simulink model "QD2_DroneStack_PID_AM32ESC_R2022b"  (R2022b)
settings: Solver=ode1  StartTime=0.0  StopTime=inf  FixedStep=1/1000  RelTol=1e-3  EnableMultiTasking=on
InitFcn:
  | Motor_Mapping_7_Inch
model workspace (MAT data in the model file):
  target_system = 1
undefined symbols (not defined in the file): _Commander, _QDrone2, _Stabilizer, datetime, HIL, KT, lf, log_, log_QD2_, m, Motor_Matrix, n, qc_get_step_size, s, saved_data
libraries: quarc_library x170, simulink x35, simulink_extras x11
(part 4 of 7)

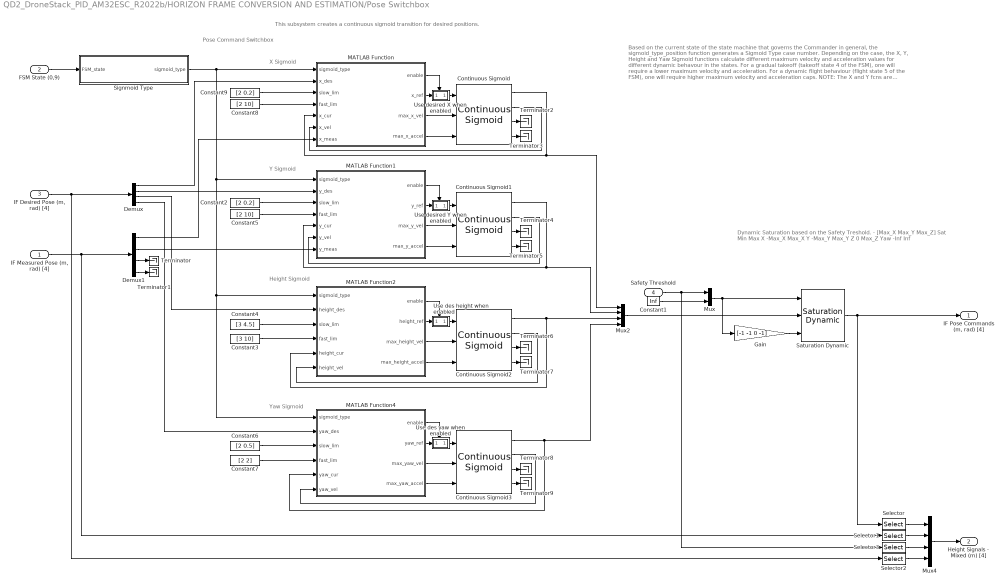
== system QD2_DroneStack_PID_AM32ESC_R2022b/HORIZON FRAME CONVERSION AND ESTIMATION/Pose Switchbox ==
  note: Dynamic Saturation based on the Safety Treshold. - [Max_X Max_Y Max_Z]
      |
      | Sat Min Max
      | X -Max_X Max_X
      | Y -Max_Y Max_Y
      | Z 0 Max_Z
      | Yaw -Inf Inf
  note: Based on the current state of the state machine that governs the Commander in general,
      | the sigmoid_type_position function generates a Sigmoid Type case number. Depending on
      | the case, the X, Y, Height and Yaw Sigmoid functions calculate different maximum velocity
      | and acceleration values for different dynamic behavour in the states.
      |
      | For a gradual takeoff (takeoff state 4 of the FSM), one will require a lower maximum velocity
      | and acceleration. For a dynamic flight behaviour (flight state 5 of the FSM), one will require
      | higher maximum velocity and acceleration caps.
      |
      | NOTE: The X and Y fcns are logically identical due to the generally symmetric X and Y behaviour.
      | The Z and Yaw fcns are different.
  note: This subsystem creates a continuous sigmoid transition for desired positions.
  note: Height Sigmoid
  note: Pose Command Switchbox
  note: X Sigmoid
  note: Yaw Sigmoid
  note: Y Sigmoid
  "IF Measured Pose (m, rad) [4]" : Inport
  FSM State (0,9) : Inport  Port=2
  "IF Desired Pose (m, rad) [4]" : Inport  Port=3
  Safety Threshold : Inport  Port=4
  Constant1 : Constant  Value=Inf
  Constant2 : Constant  Value=[2 0.2]
  Constant3 : Constant  Value=[3 10]
  Constant4 : Constant  Value=[3 4.5]
  Constant5 : Constant  Value=[2 10]
  Constant6 : Constant  Value=[2 0.5]
  Constant7 : Constant  Value=[2 2]
  Constant8 : Constant  Value=[2 10]
  Constant9 : Constant  Value=[2 0.2]
  Continuous Sigmoid{,1..3} (4 alike) : quarc_library/Sources/Sigmoids/Continuous Sigmoid  params_source=External (input ports)  max_velocity=2  max_acceleration=10  initial_position=0  initial_velocity=0  hold_off=0.5  input_sample_time=-1  output_sample_time=qc_get_step_size
      settings: SourceProductName=QUARC Targets
  Demux : Demux
  Demux1 : Demux
  Gain : Gain  Gain=[-1 -1 0 -1]
  MATLAB Function : MATLAB Function  TreatAsAtomicUnit=on
  MATLAB Function1 : MATLAB Function  TreatAsAtomicUnit=on
  MATLAB Function2 : MATLAB Function  TreatAsAtomicUnit=on
  MATLAB Function4 : MATLAB Function  TreatAsAtomicUnit=on
  Mux : Mux  Inputs=2
  Mux2 : Mux
  Mux4 : Mux
  Saturation Dynamic : simulink/Discontinuities/Saturation Dynamic  OutMin=[]  OutMax=[]  OutDataTypeStr=Inherit: Same as second input  OutDataType=fixdt(1, 16)  OutScaling=2^-10  DoSatur=off
  Selector : Selector  InputPortWidth=4  IndexOptions=Index vector (dialog)  Indices=[3]  OutputSizes=1
  Selector1 : Selector  InputPortWidth=4  IndexOptions=Index vector (dialog)  Indices=[3]  OutputSizes=1
  Selector2 : Selector  InputPortWidth=4  IndexOptions=Index vector (dialog)  Indices=[3]  OutputSizes=1
  Selector3 : Selector  InputPortWidth=3  IndexOptions=Index vector (dialog)  Indices=[3]  OutputSizes=1
  Signmoid Type : MATLAB Function  TreatAsAtomicUnit=on
  Terminator{,1..9} (10 alike) : Terminator
  Use des height when enabled : Subsystem  TreatAsAtomicUnit=on
  Use des yaw when enabled : Subsystem  TreatAsAtomicUnit=on
  Use desired X when enabled : Subsystem  TreatAsAtomicUnit=on
  Use desired Y when enabled : Subsystem  TreatAsAtomicUnit=on
  "IF Pose Commands (m, rad) [4]" : Outport  VectorParamsAs1DForOutWhenUnconnected=off
  Height Signals - Mixed (m) [4] : Outport  Port=2  VectorParamsAs1DForOutWhenUnconnected=off
  wires:
  Constant4/1 -> MATLAB Function2/3(slow_lim)
  Constant3/1 -> MATLAB Function2/4(fast_lim)
  Selector/1 -> Mux4/1
  Selector1/1 -> Mux4/2
  Selector2/1 -> Mux4/4
  Selector3/1 -> Mux4/3
  Safety Threshold/1 -> Mux/1, Selector3/1
  Mux/1 -> Saturation Dynamic/1, Gain/1
  Constant1/1 -> Mux/2
  Saturation Dynamic/1 -> "IF Pose Commands (m, rad) [4]"/1, Selector/1
  Mux2/1 -> Saturation Dynamic/2
  Mux4/1 -> Height Signals - Mixed (m) [4]/1
  Gain/1 -> Saturation Dynamic/3
  Demux/2 -> MATLAB Function1/2(y_des)
  Use desired Y when enabled/1(Out1) -> Continuous Sigmoid1/1
  Use desired X when enabled/1(Out1) -> Continuous Sigmoid/1
  MATLAB Function2/3(max_height_vel) -> Continuous Sigmoid2/2
  Continuous Sigmoid3/3 -> Terminator8/1
  Demux1/4 -> Terminator1/1
  MATLAB Function4/1(enable) -> Use des yaw when enabled/Enable
  Use des yaw when enabled/1(Out1) -> Continuous Sigmoid3/1
  Continuous Sigmoid1/2 -> MATLAB Function1/6(y_vel)
  Constant2/1 -> MATLAB Function1/3(slow_lim)
  Constant6/1 -> MATLAB Function4/3(slow_lim)
  Demux1/1 -> MATLAB Function/7(x_meas)
  MATLAB Function1/2(y_ref) -> Use desired Y when enabled/1(h_d (m) [1])
  Demux/3 -> MATLAB Function2/2(height_des)
  Constant7/1 -> MATLAB Function4/4(fast_lim)
  Continuous Sigmoid1/4 -> Terminator5/1
  MATLAB Function1/1(enable) -> Use desired Y when enabled/Enable
  Continuous Sigmoid2/4 -> Terminator7/1
  Demux1/3 -> Terminator/1
  Signmoid Type/1(sigmoid_type) -> MATLAB Function/1(sigmoid_type), MATLAB Function1/1(sigmoid_type), MATLAB Function2/1(sigmoid_type), MATLAB Function4/1(sigmoid_type)
  MATLAB Function/3(max_x_vel) -> Continuous Sigmoid/2
  MATLAB Function2/1(enable) -> Use des height when enabled/Enable
  Constant9/1 -> MATLAB Function/3(slow_lim)
  Continuous Sigmoid2/2 -> MATLAB Function2/6(height_vel)
  Continuous Sigmoid1/1 -> MATLAB Function1/5(y_cur), Mux2/2
  MATLAB Function4/4(max_yaw_accel) -> Continuous Sigmoid3/3
  Demux/1 -> MATLAB Function/2(x_des)
  MATLAB Function1/3(max_y_vel) -> Continuous Sigmoid1/2
  Continuous Sigmoid3/2 -> MATLAB Function4/6(yaw_vel)
  MATLAB Function2/2(height_ref) -> Use des height when enabled/1(h_d (m) [1])
  MATLAB Function/4(max_x_accel) -> Continuous Sigmoid/3
  Use des height when enabled/1(Out1) -> Continuous Sigmoid2/1
  Continuous Sigmoid2/3 -> Terminator6/1
  Demux/4 -> MATLAB Function4/2(yaw_des)
  MATLAB Function1/4(max_y_accel) -> Continuous Sigmoid1/3
  MATLAB Function/1(enable) -> Use desired X when enabled/Enable
  Continuous Sigmoid3/4 -> Terminator9/1
  MATLAB Function4/2(yaw_ref) -> Use des yaw when enabled/1(h_d (m) [1])
  FSM State (0,9)/1 -> Signmoid Type/1(FSM_state)
  MATLAB Function2/4(max_height_accel) -> Continuous Sigmoid2/3
  Continuous Sigmoid/4 -> Terminator3/1
  Continuous Sigmoid/3 -> Terminator2/1
  Continuous Sigmoid/1 -> MATLAB Function/5(x_cur), Mux2/1
  Continuous Sigmoid/2 -> MATLAB Function/6(x_vel)
  MATLAB Function/2(x_ref) -> Use desired X when enabled/1(h_d (m) [1])
  Continuous Sigmoid3/1 -> MATLAB Function4/5(yaw_cur), Mux2/4
  MATLAB Function4/3(max_yaw_vel) -> Continuous Sigmoid3/2
  Continuous Sigmoid2/1 -> MATLAB Function2/5(height_cur), Mux2/3
  Demux1/2 -> MATLAB Function1/7(y_meas)
  Continuous Sigmoid1/3 -> Terminator4/1
  "IF Measured Pose (m, rad) [4]"/1 -> Demux1/1, Selector1/1
  "IF Desired Pose (m, rad) [4]"/1 -> Demux/1, Selector2/1
  Constant5/1 -> MATLAB Function1/4(fast_lim)
  Constant8/1 -> MATLAB Function/4(fast_lim)

== system QD2_DroneStack_PID_AM32ESC_R2022b/QDrone 2 DAQ/Attitude Estimate from IMU Data ==
  IMU Data [12] : Inport
  For Each Subsystem - Iterate over IMU0 and IMU1 : Subsystem  TreatAsAtomicUnit=on
  Reshape into 2 columns for IMU0 and IMU1 : Reshape  OutputDimensionality=Customize  OutputDimensions=[6,2]
  Select Data for IMU0 : Selector  NumberOfDimensions=2  InputPortWidth=3  IndexOptions=Index vector (dialog),Index vector (dialog)  Indices=[1:9],[1]  OutputSizes=1,1
  Select Data for IMU1 : Selector  NumberOfDimensions=2  InputPortWidth=3  IndexOptions=Index vector (dialog),Index vector (dialog)  Indices=[1:9],[2]  OutputSizes=1,1
  "BF Estimated Attitude for IMU0 (rad, rad/s, rad/2^2) [9]" : Outport
  "BF Estimated Attitude for IMU1 (rad, rad/s, rad/2^2) [9]" : Outport  Port=2
  wires:
  IMU Data [12]/1 -> Reshape into 2 columns for IMU0 and IMU1/1
  Reshape into 2 columns for IMU0 and IMU1/1 -> For Each Subsystem - Iterate over IMU0 and IMU1/1(IMU Data [6xn])
  For Each Subsystem - Iterate over IMU0 and IMU1/1("BF Estimated Attitude (rad, rad/s, rad/2^2) [9xn]") -> Select Data for IMU1/1, Select Data for IMU0/1
  Select Data for IMU0/1 -> "BF Estimated Attitude for IMU0 (rad, rad/s, rad/2^2) [9]"/1
  Select Data for IMU1/1 -> "BF Estimated Attitude for IMU1 (rad, rad/s, rad/2^2) [9]"/1

== system QD2_DroneStack_PID_AM32ESC_R2022b/QDrone 2 DAQ/Choose Motor Telemetry ==
  enable telemetry : Inport
  Bias1 : Bias  Bias=0:3  SaturateOnIntegerOverflow=off
  Constant1 : Constant  Value="[0 0 0 0; 1 0 0 0; 0 0 0 0; 0 1 0 0; 0 0 0 0; 0 0 1 0; 0 0 0 0;  0 0 0 1]"
  Constant2 : Constant  Value=8
  Gain : Gain  Gain=.7
  MATLAB Function : MATLAB Function  TreatAsAtomicUnit=on
  Selector : Selector  NumberOfDimensions=2  IndexMode=Zero-based  InputPortWidth=3  IndexOptions=Index vector (port),Select all  Indices=[1 3],1  OutputSizes=1,1
  Telemetry : Scope
  Zero-Order Hold1 : ZeroOrderHold  SampleTime=-1
  Motor telemetry select : Outport
  Motor telemetry index : Outport  Port=2
  wires:
  Gain/1 -> Bias1/1
  Bias1/1 -> Telemetry/1
  MATLAB Function/1(idx) -> Zero-Order Hold1/1
  Zero-Order Hold1/1 -> Selector/2, Motor telemetry index/1
  enable telemetry/1 -> MATLAB Function/1(enable)
  Selector/1 -> Motor telemetry select/1, Gain/1
  Constant1/1 -> Selector/1
  Constant2/1 -> MATLAB Function/2(n)

== system QD2_DroneStack_PID_AM32ESC_R2022b/QDrone 2 DAQ/Construct ESC Speed ==
  ESC Data In [4] : Inport
  ESC Channel Select : Inport  Port=2
  For Each Subsystem - Construct ESC Signal : Subsystem  TreatAsAtomicUnit=on
  Memory : Memory  InitialCondition=zeros(1,4)
  ESC Data Out [4] : Outport
  wires:
  For Each Subsystem - Construct ESC Signal/1(ESC Data Out [4]) -> ESC Data Out [4]/1, Memory/1
  Memory/1 -> For Each Subsystem - Construct ESC Signal/3(ESC Previous Data [4])
  ESC Data In [4]/1 -> For Each Subsystem - Construct ESC Signal/1(ESC Data In [4])
  ESC Channel Select/1 -> For Each Subsystem - Construct ESC Signal/2(ESC Channel)

== system QD2_DroneStack_PID_AM32ESC_R2022b/QDrone 2 DAQ/Construct ESC Temperature ==
  ESC Data In [4] : Inport
  ESC Channel Select : Inport  Port=2
  For Each Subsystem - Construct ESC Signal : Subsystem  TreatAsAtomicUnit=on
  Memory : Memory  InitialCondition=zeros(1,4)
  ESC Data Out [4] : Outport
  wires:
  For Each Subsystem - Construct ESC Signal/1(ESC Data Out [4]) -> ESC Data Out [4]/1, Memory/1
  Memory/1 -> For Each Subsystem - Construct ESC Signal/3(ESC Previous Data [4])
  ESC Data In [4]/1 -> For Each Subsystem - Construct ESC Signal/1(ESC Data In [4])
  ESC Channel Select/1 -> For Each Subsystem - Construct ESC Signal/2(ESC Channel)

== system QD2_DroneStack_PID_AM32ESC_R2022b/QDrone 2 DAQ/Construct ESC Voltage ==
  ESC Data In [4] : Inport
  ESC Channel Select : Inport  Port=2
  For Each Subsystem - Construct ESC Signal : Subsystem  TreatAsAtomicUnit=on
  Memory : Memory  InitialCondition=zeros(1,4)
  ESC Data Out [4] : Outport
  wires:
  ESC Channel Select/1 -> For Each Subsystem - Construct ESC Signal/2(ESC Channel)
  ESC Data In [4]/1 -> For Each Subsystem - Construct ESC Signal/1(ESC Data In [4])
  Memory/1 -> For Each Subsystem - Construct ESC Signal/3(ESC Previous Data [4])
  For Each Subsystem - Construct ESC Signal/1(ESC Data Out [4]) -> Memory/1, ESC Data Out [4]/1

== system QD2_DroneStack_PID_AM32ESC_R2022b/QDrone 2 DAQ/Detect ESC Problems ==
  ESC Telemetry Enabled : Inport
  ESC Channel Request [4] : Inport  Port=2
  ESC Channel Reported [4] : Inport  Port=3
  AND : Logic  IconShape=distinctive  AllPortsSameDT=off  OutDataTypeStr=boolean
  Compare To Constant : simulink/Logic and Bit Operations/Compare To Constant  relop=>=  const=20  OutDataTypeStr=boolean
  Constant : Constant  Value=200
  Delay{,1..3} (4 alike) : Delay
  Demux{,1..2,8} (4 alike) : Demux
  ESC Channel Mismatrch : Scope  NumInputPorts=4
  ESC Channel Mismatrch Count : Scope  NumInputPorts=4
  ESC Channel Selection Index : Scope  NumInputPorts=4
  For Each Subsystem : Subsystem  TreatAsAtomicUnit=on
  MATLAB Function : MATLAB Function  TreatAsAtomicUnit=on
  Mux : Mux
  Mux{1..4} (4 alike) : Mux  Inputs=2
  ESC Comm Problem [4] : Outport
  wires:
  ESC Channel Reported [4]/1 -> Demux2/1, For Each Subsystem/2(Channel Reported [4])
  Demux/1 -> Delay3/1
  Demux/2 -> Delay2/1
  Demux/3 -> Delay1/1
  Demux/4 -> Delay/1
  ESC Channel Request [4]/1 -> Demux/1
  Delay2/1 -> Mux2/1, Mux/2
  Delay3/1 -> Mux/1, Mux1/1
  Delay1/1 -> Mux3/1, Mux/3
  Delay/1 -> Mux4/1, Mux/4
  Mux/1 -> For Each Subsystem/1(Channel Requested [4])
  For Each Subsystem/1(mismatched [4]) -> AND/1
  AND/1 -> MATLAB Function/1(u), Demux8/1
  Demux8/2 -> ESC Channel Mismatrch/3
  Demux8/1 -> ESC Channel Mismatrch/4
  Demux8/3 -> ESC Channel Mismatrch/2
  Demux8/4 -> ESC Channel Mismatrch/1
  Constant/1 -> MATLAB Function/2(buffer_size)
  Demux1/4 -> ESC Channel Mismatrch Count/1
  Demux1/3 -> ESC Channel Mismatrch Count/2
  Demux1/1 -> ESC Channel Mismatrch Count/4
  Demux1/2 -> ESC Channel Mismatrch Count/3
  MATLAB Function/1(n) -> Compare To Constant/1, Demux1/1
  Compare To Constant/1 -> ESC Comm Problem [4]/1
  ESC Telemetry Enabled/1 -> AND/2
  Demux2/1 -> Mux1/2
  Demux2/2 -> Mux2/2
  Demux2/3 -> Mux3/2
  Demux2/4 -> Mux4/2
  Mux4/1 -> ESC Channel Selection Index/1
  Mux3/1 -> ESC Channel Selection Index/2
  Mux2/1 -> ESC Channel Selection Index/3
  Mux1/1 -> ESC Channel Selection Index/4

== system QD2_DroneStack_PID_AM32ESC_R2022b/QDrone 2 DAQ/Enabled Subsystem - Write ESC Commands ==
  DShot Raw [4] : Inport
  Enable : EnablePort
  HIL Write PWM : quarc_library/Data Acquisition/Generic/Immediate I//O/HIL Write PWM  object_name=HIL-1  channels=[0:3]  sample_time=-1  active=off  vector_input=on
      settings: AttributesFormatString=(%<object_name>)  SourceProductName=QUARC Targets
  wires:
  DShot Raw [4]/1 -> HIL Write PWM/1

== system QD2_DroneStack_PID_AM32ESC_R2022b/QDrone 2 DAQ/Generate LED Pattern ==
  ESC States : Inport
  Blue Blue : Constant  Value=[0 0 1 0 0 1]
  Green Green : Constant  Value=[0 1 0 0 1 0]
  LED OFF : Constant  Value=[ 0 0 0 0 0 0]
  Multiport Switch : MultiPortSwitch  DataPortOrder=Specify indices  DataPortIndices={0,1,2,3,4,5,77,88,99}  DataPortForDefault=Additional data port  DiagnosticForDefault=Warning  SaturateOnIntegerOverflow=off  InputSameDT=off
  Red Blue : Constant  Value="[ 1 0 0 0 0 1   ]"
  Red Red : Constant  Value=[ 1 0 0 1 0 0]
  Red Yellow : Constant  Value="[ 1 0 0 1 1 0  ]"
  Yellow Blue : Constant  Value="[ 1 1 0 0 0 1  ]"
  Yellow Green : Constant  Value="[ 1 1 0 0 1 0  ]"
  Yellow Red : Constant  Value="[ 1 1 0 1 0 0  ]"
  Yellow Yellow : Constant  Value="[ 1 1 0 1 1 0  ]"
  LED Command : Outport
  wires:
  Multiport Switch/1 -> LED Command/1
  ESC States/1 -> Multiport Switch/1
  Blue Blue/1 -> Multiport Switch/4
  Red Red/1 -> Multiport Switch/10
  Yellow Yellow/1 -> Multiport Switch/2
  Red Blue/1 -> Multiport Switch/9
  Yellow Blue/1 -> Multiport Switch/8
  LED OFF/1 -> Multiport Switch/11
  Green Green/1 -> Multiport Switch/7
  Yellow Green/1 -> Multiport Switch/3
  Yellow Red/1 -> Multiport Switch/5
  Red Yellow/1 -> Multiport Switch/6

== system QD2_DroneStack_PID_AM32ESC_R2022b/QDrone 2 DAQ/Monitor Battery Level ==
  note: Monitor Battery Level.
      | Flag Low Battery Error if
      | Battery level dips below
      | threshold for specified
      | threshold time period.
  Battery (V) : Inport
  AND : Logic  IconShape=distinctive  AllPortsSameDT=off  OutDataTypeStr=boolean
  Battery Low Time Threshold (s) : Constant  Value=0.3
  Constant : Constant  Value=0.5
  Data Type Conversion : DataTypeConversion  SaturateOnIntegerOverflow=off  RndMeth=Floor
  Data Type Conversion1 : DataTypeConversion  SaturateOnIntegerOverflow=off  RndMeth=Floor
  Greater than minimum expected voltage (Valid Battery Reading) : simulink/Logic and Bit Operations/Compare To Constant  relop=>  const=0.5  OutDataTypeStr=boolean
  Less than minimum threshold voltage (Battery level too low) : simulink/Logic and Bit Operations/Compare To Constant  relop=<=  const=14  OutDataTypeStr=boolean
  Terminator : Terminator
  Threshold : quarc_library/Discontinuities/Threshold  operator=>=  param_src=External input port  threshold=0  duration=0
      settings: SourceProductName=QUARC Targets
  Triggered Subsystem - Latching Flag : Subsystem  TreatAsAtomicUnit=on
  Low Battery : Outport
  wires:
  Battery (V)/1 -> Less than minimum threshold voltage (Battery level too low)/1, Greater than minimum expected voltage (Valid Battery Reading)/1
  Less than minimum threshold voltage (Battery level too low)/1 -> AND/2
  Greater than minimum expected voltage (Valid Battery Reading)/1 -> AND/1
  AND/1 -> Data Type Conversion/1
  Constant/1 -> Threshold/2
  Battery Low Time Threshold (s)/1 -> Threshold/3
  Data Type Conversion/1 -> Threshold/1
  Threshold/2 -> Terminator/1
  Threshold/1 -> Triggered Subsystem - Latching Flag/Trigger
  Triggered Subsystem - Latching Flag/1(Out1) -> Data Type Conversion1/1
  Data Type Conversion1/1 -> Low Battery/1

== system QD2_DroneStack_PID_AM32ESC_R2022b/QDrone 2 DAQ/Sensor Failure Monitoring ==
  note: Check if any of the IMU signal lines have "flatlined"
      | i.e., remain at exactly 0 value for 1 second or more
  IMU Data [12] : Inport
  Model Time : Inport  Port=2
  AND : Logic  IconShape=distinctive  AllPortsSameDT=off  OutDataTypeStr=boolean
  Compare : quarc_library/Logic Operations/Compare  operator=>=  output_data_type=boolean
      settings: SourceProductName=QUARC Targets
  Constant1 : Constant
  Constant2 : Constant  Value=0
  Demux : Demux  Outputs=12
  OR : Logic  Operator=OR  Inputs=12  AllPortsSameDT=off  OutDataTypeStr=boolean
  Terminator{,1..11} (12 alike) : Terminator
  Threshold{,1..11} (12 alike) : quarc_library/Discontinuities/Threshold  operator===  param_src=External input port  threshold=0  duration=1
      settings: SourceProductName=QUARC Targets
  Sensor Fault : Outport
  wires:
  Model Time/1 -> Compare/1
  Constant1/1 -> Threshold1/3, Threshold2/3, Threshold3/3, Threshold5/3, Threshold6/3, Threshold7/3, Threshold8/3, Threshold9/3, Threshold10/3, Threshold11/3, Threshold4/3, Threshold/3, Compare/2
  Demux/1 -> Threshold/1
  Demux/2 -> Threshold1/1
  Constant2/1 -> Threshold1/2, Threshold2/2, Threshold3/2, Threshold4/2, Threshold5/2, Threshold6/2, Threshold7/2, Threshold8/2, Threshold9/2, Threshold10/2, Threshold11/2, Threshold/2
  IMU Data [12]/1 -> Demux/1
  Demux/3 -> Threshold2/1
  Demux/4 -> Threshold3/1
  Demux/5 -> Threshold4/1
  Demux/6 -> Threshold5/1
  Demux/7 -> Threshold6/1
  Demux/8 -> Threshold7/1
  Demux/9 -> Threshold8/1
  Demux/10 -> Threshold9/1
  Demux/11 -> Threshold10/1
  Demux/12 -> Threshold11/1
  Threshold/1 -> OR/1
  Threshold1/1 -> OR/2
  Threshold2/1 -> OR/3
  Threshold3/1 -> OR/4
  Threshold4/1 -> OR/5
  Threshold5/1 -> OR/6
  Threshold6/1 -> OR/7
  Threshold7/1 -> OR/8
  Threshold8/1 -> OR/9
  Threshold9/1 -> OR/10
  Threshold10/1 -> OR/11
  Threshold11/1 -> OR/12
  Threshold/2 -> Terminator/1
  Threshold1/2 -> Terminator1/1
  Threshold2/2 -> Terminator2/1
  Threshold3/2 -> Terminator3/1
  Threshold4/2 -> Terminator4/1
  Threshold5/2 -> Terminator5/1
  Threshold6/2 -> Terminator6/1
  Threshold7/2 -> Terminator7/1
  Threshold8/2 -> Terminator8/1
  Threshold9/2 -> Terminator9/1
  Threshold10/2 -> Terminator10/1
  Threshold11/2 -> Terminator11/1
  Compare/1 -> AND/1
  OR/1 -> AND/2
  AND/1 -> Sensor Fault/1

== system QD2_DroneStack_PID_AM32ESC_R2022b/QDrone 2 DAQ/Timing Monitors ==
  note: Base Model Rate (1kHz)
  note: Optical Flow Rate (100 Hz)
  note: ToF Range Rate (25 Hz)
  Computation Time : quarc_library/Sources/Time/Computation Time  sample_time=qc_get_step_size  use_model=on  use_cpu_time=off
  Computation Time1 : quarc_library/Sources/Time/Computation Time  sample_time=0.01  use_model=on  use_cpu_time=off
  Computation Time2 : quarc_library/Sources/Time/Computation Time  sample_time=0.04  use_model=on  use_cpu_time=off
  Mux : Mux  Inputs=2
  Mux1 : Mux  Inputs=2
  Mux2 : Mux  Inputs=2
  Mux3 : Mux  Inputs=3
  Rate Transition{,1..3} (4 alike) : RateTransition
  Sample Time : quarc_library/Sources/Time/Sample Time  Priority=-99  sample_time=qc_get_step_size
  Sample Time1 : quarc_library/Sources/Time/Sample Time  Priority=-99  sample_time=0.01
  Sample Time2 : quarc_library/Sources/Time/Sample Time  Priority=-99  sample_time=0.04
  Timing Check : Scope  NumInputPorts=3
  Timings : Outport
  wires:
  Computation Time/1 -> Mux/1
  Sample Time/1 -> Mux/2
  Sample Time1/1 -> Rate Transition1/1
  Computation Time1/1 -> Rate Transition/1
  Computation Time2/1 -> Rate Transition2/1
  Sample Time2/1 -> Rate Transition3/1
  Mux1/1 -> Mux3/2, Timing Check/2
  Mux/1 -> Timing Check/1, Mux3/1
  Mux2/1 -> Timing Check/3, Mux3/3
  Mux3/1 -> Timings/1
  Rate Transition/1 -> Mux1/1
  Rate Transition1/1 -> Mux1/2
  Rate Transition2/1 -> Mux2/1
  Rate Transition3/1 -> Mux2/2

== system QD2_DroneStack_PID_AM32ESC_R2022b/QDrone 2 DAQ - OLD/Attitude Estimate from IMU Data ==
  IMU Data [12] : Inport
  For Each Subsystem - Iterate over IMU0 and IMU1 : Subsystem  TreatAsAtomicUnit=on
  Reshape into 2 columns for IMU0 and IMU1 : Reshape  OutputDimensionality=Customize  OutputDimensions=[6,2]
  Select Data for IMU0 : Selector  NumberOfDimensions=2  InputPortWidth=3  IndexOptions=Index vector (dialog),Index vector (dialog)  Indices=[1:9],[1]  OutputSizes=1,1
  Select Data for IMU1 : Selector  NumberOfDimensions=2  InputPortWidth=3  IndexOptions=Index vector (dialog),Index vector (dialog)  Indices=[1:9],[2]  OutputSizes=1,1
  "BF Estimated Attitude for IMU0 (rad, rad/s, rad/2^2) [9]" : Outport
  "BF Estimated Attitude for IMU1 (rad, rad/s, rad/2^2) [9]" : Outport  Port=2
  wires:
  IMU Data [12]/1 -> Reshape into 2 columns for IMU0 and IMU1/1
  Reshape into 2 columns for IMU0 and IMU1/1 -> For Each Subsystem - Iterate over IMU0 and IMU1/1(IMU Data [6xn])
  For Each Subsystem - Iterate over IMU0 and IMU1/1("BF Estimated Attitude (rad, rad/s, rad/2^2) [9xn]") -> Select Data for IMU1/1, Select Data for IMU0/1
  Select Data for IMU0/1 -> "BF Estimated Attitude for IMU0 (rad, rad/s, rad/2^2) [9]"/1
  Select Data for IMU1/1 -> "BF Estimated Attitude for IMU1 (rad, rad/s, rad/2^2) [9]"/1

== system QD2_DroneStack_PID_AM32ESC_R2022b/QDrone 2 DAQ - OLD/Choose Motor Telemetry ==
  enable telemetry : Inport
  Bias1 : Bias  Bias=0:3  SaturateOnIntegerOverflow=off
  Constant1 : Constant  Value=[0 0 0 0; 0 0 0 1; 0 0 0 0; 0 0 1 0; 0 0 0 0; 0 1 0 0; 0 0 0 0; 1 0 0 0]
  Constant2 : Constant  Value=8
  Gain : Gain  Gain=.7
  MATLAB Function : MATLAB Function  TreatAsAtomicUnit=on
  Selector : Selector  NumberOfDimensions=2  IndexMode=Zero-based  InputPortWidth=3  IndexOptions=Index vector (port),Select all  Indices=[1 3],1  OutputSizes=1,1
  Telemetry : Scope
  Zero-Order Hold1 : ZeroOrderHold  SampleTime=-1
  Motor telemetry select : Outport
  Motor telemetry index : Outport  Port=2
  wires:
  Gain/1 -> Bias1/1
  Bias1/1 -> Telemetry/1
  MATLAB Function/1(idx) -> Zero-Order Hold1/1
  Zero-Order Hold1/1 -> Selector/2, Motor telemetry index/1
  enable telemetry/1 -> MATLAB Function/1(enable)
  Selector/1 -> Motor telemetry select/1, Gain/1
  Constant1/1 -> Selector/1
  Constant2/1 -> MATLAB Function/2(n)

== system QD2_DroneStack_PID_AM32ESC_R2022b/QDrone 2 DAQ - OLD/Construct ESC Speed ==
  ESC Data In [4] : Inport
  ESC Channel Select : Inport  Port=2
  For Each Subsystem - Construct ESC Signal : Subsystem  TreatAsAtomicUnit=on
  Memory : Memory  InitialCondition=zeros(1,4)
  ESC Data Out [4] : Outport
  wires:
  For Each Subsystem - Construct ESC Signal/1(ESC Data Out [4]) -> ESC Data Out [4]/1, Memory/1
  Memory/1 -> For Each Subsystem - Construct ESC Signal/3(ESC Previous Data [4])
  ESC Data In [4]/1 -> For Each Subsystem - Construct ESC Signal/1(ESC Data In [4])
  ESC Channel Select/1 -> For Each Subsystem - Construct ESC Signal/2(ESC Channel)

== system QD2_DroneStack_PID_AM32ESC_R2022b/QDrone 2 DAQ - OLD/Construct ESC Temperature ==
  ESC Data In [4] : Inport
  ESC Channel Select : Inport  Port=2
  For Each Subsystem - Construct ESC Signal : Subsystem  TreatAsAtomicUnit=on
  Memory : Memory  InitialCondition=zeros(1,4)
  ESC Data Out [4] : Outport
  wires:
  For Each Subsystem - Construct ESC Signal/1(ESC Data Out [4]) -> ESC Data Out [4]/1, Memory/1
  Memory/1 -> For Each Subsystem - Construct ESC Signal/3(ESC Previous Data [4])
  ESC Data In [4]/1 -> For Each Subsystem - Construct ESC Signal/1(ESC Data In [4])
  ESC Channel Select/1 -> For Each Subsystem - Construct ESC Signal/2(ESC Channel)

== system QD2_DroneStack_PID_AM32ESC_R2022b/QDrone 2 DAQ - OLD/Construct ESC Voltage ==
  ESC Data In [4] : Inport
  ESC Channel Select : Inport  Port=2
  For Each Subsystem - Construct ESC Signal : Subsystem  TreatAsAtomicUnit=on
  Memory : Memory  InitialCondition=zeros(1,4)
  ESC Data Out [4] : Outport
  wires:
  ESC Channel Select/1 -> For Each Subsystem - Construct ESC Signal/2(ESC Channel)
  ESC Data In [4]/1 -> For Each Subsystem - Construct ESC Signal/1(ESC Data In [4])
  Memory/1 -> For Each Subsystem - Construct ESC Signal/3(ESC Previous Data [4])
  For Each Subsystem - Construct ESC Signal/1(ESC Data Out [4]) -> Memory/1, ESC Data Out [4]/1

== system QD2_DroneStack_PID_AM32ESC_R2022b/QDrone 2 DAQ - OLD/Detect ESC Problems ==
  ESC Telemetry Enabled : Inport
  ESC Channel Request [4] : Inport  Port=2
  ESC Channel Reported [4] : Inport  Port=3
  AND : Logic  IconShape=distinctive  AllPortsSameDT=off  OutDataTypeStr=boolean
  Compare To Constant : simulink/Logic and Bit Operations/Compare To Constant  relop=>=  const=10  OutDataTypeStr=boolean
  Constant : Constant  Value=100
  Delay{,1..3} (4 alike) : Delay
  Demux : Demux
  Demux1 : Demux
  Demux8 : Demux
  ESC Channel Mismatrch : Scope  NumInputPorts=4
  ESC Channel Mismatrch Count : Scope  NumInputPorts=4
  For Each Subsystem : Subsystem  TreatAsAtomicUnit=on
  MATLAB Function : MATLAB Function  TreatAsAtomicUnit=on
  Mux : Mux
  ESC Comm Problem [4] : Outport
  wires:
  ESC Channel Reported [4]/1 -> For Each Subsystem/2(Channel Reported [4])
  Demux/1 -> Delay3/1
  Demux/2 -> Delay2/1
  Demux/3 -> Delay1/1
  Demux/4 -> Delay/1
  ESC Channel Request [4]/1 -> Demux/1
  Delay2/1 -> Mux/2
  Delay3/1 -> Mux/1
  Delay1/1 -> Mux/3
  Delay/1 -> Mux/4
  Mux/1 -> For Each Subsystem/1(Channel Requested [4])
  For Each Subsystem/1(mismatched [4]) -> AND/1
  AND/1 -> MATLAB Function/1(u), Demux8/1
  Demux8/2 -> ESC Channel Mismatrch/3
  Demux8/1 -> ESC Channel Mismatrch/4
  Demux8/3 -> ESC Channel Mismatrch/2
  Demux8/4 -> ESC Channel Mismatrch/1
  Constant/1 -> MATLAB Function/2(buffer_size)
  Demux1/4 -> ESC Channel Mismatrch Count/1
  Demux1/3 -> ESC Channel Mismatrch Count/2
  Demux1/1 -> ESC Channel Mismatrch Count/4
  Demux1/2 -> ESC Channel Mismatrch Count/3
  MATLAB Function/1(n) -> Compare To Constant/1, Demux1/1
  Compare To Constant/1 -> ESC Comm Problem [4]/1
  ESC Telemetry Enabled/1 -> AND/2

== system QD2_DroneStack_PID_AM32ESC_R2022b/QDrone 2 DAQ - OLD/Enabled Subsystem - Write ESC Commands ==
  DShot Raw [4] : Inport
  Enable : EnablePort
  HIL Write PWM : quarc_library/Data Acquisition/Generic/Immediate I//O/HIL Write PWM  object_name=HIL-1  channels=[0:3]  sample_time=-1  active=off  vector_input=on
      settings: AttributesFormatString=(%<object_name>)  SourceProductName=QUARC Targets
  wires:
  DShot Raw [4]/1 -> HIL Write PWM/1

== system QD2_DroneStack_PID_AM32ESC_R2022b/QDrone 2 DAQ - OLD/Generate LED Pattern ==
  ESC States : Inport
  Blue Blue : Constant  Value=[0 0 1 0 0 1]
  Green Green : Constant  Value=[0 1 0 0 1 0]
  LED OFF : Constant  Value=[ 0 0 0 0 0 0]
  Multiport Switch : MultiPortSwitch  DataPortOrder=Specify indices  DataPortIndices={0,1,2,3,4,5,77,88,99}  DataPortForDefault=Additional data port  DiagnosticForDefault=Warning  SaturateOnIntegerOverflow=off  InputSameDT=off
  Red Blue : Constant  Value="[ 1 0 0 0 0 1   ]"
  Red Red : Constant  Value=[ 1 0 0 1 0 0]
  Red Yellow : Constant  Value="[ 1 0 0 1 1 0  ]"
  Yellow Blue : Constant  Value="[ 1 1 0 0 0 1  ]"
  Yellow Green : Constant  Value="[ 1 1 0 0 1 0  ]"
  Yellow Red : Constant  Value="[ 1 1 0 1 0 0  ]"
  Yellow Yellow : Constant  Value="[ 1 1 0 1 1 0  ]"
  LED Command : Outport
  wires:
  Multiport Switch/1 -> LED Command/1
  ESC States/1 -> Multiport Switch/1
  Blue Blue/1 -> Multiport Switch/4
  Red Red/1 -> Multiport Switch/10
  Yellow Yellow/1 -> Multiport Switch/2
  Red Blue/1 -> Multiport Switch/9
  Yellow Blue/1 -> Multiport Switch/8
  LED OFF/1 -> Multiport Switch/11
  Green Green/1 -> Multiport Switch/7
  Yellow Green/1 -> Multiport Switch/3
  Yellow Red/1 -> Multiport Switch/5
  Red Yellow/1 -> Multiport Switch/6

== system QD2_DroneStack_PID_AM32ESC_R2022b/QDrone 2 DAQ - OLD/Monitor Battery Level ==
  note: Monitor Battery Level.
      | Flag Low Battery Error if
      | Battery level dips below
      | threshold for specified
      | threshold time period.
  Battery (V) : Inport
  AND : Logic  IconShape=distinctive  AllPortsSameDT=off  OutDataTypeStr=boolean
  Battery Low Time Threshold (s) : Constant  Value=0.3
  Constant : Constant  Value=0.5
  Data Type Conversion : DataTypeConversion  SaturateOnIntegerOverflow=off  RndMeth=Floor
  Data Type Conversion1 : DataTypeConversion  SaturateOnIntegerOverflow=off  RndMeth=Floor
  Greater than minimum expected voltage (Valid Battery Reading) : simulink/Logic and Bit Operations/Compare To Constant  relop=>  const=0.5  OutDataTypeStr=boolean
  Less than minimum threshold voltage (Battery level too low) : simulink/Logic and Bit Operations/Compare To Constant  relop=<=  const=14  OutDataTypeStr=boolean
  Terminator : Terminator
  Threshold : quarc_library/Discontinuities/Threshold  operator=>=  param_src=External input port  threshold=0  duration=0
      settings: SourceProductName=QUARC Targets
  Triggered Subsystem - Latching Flag : Subsystem  TreatAsAtomicUnit=on
  Low Battery : Outport
  wires:
  Battery (V)/1 -> Less than minimum threshold voltage (Battery level too low)/1, Greater than minimum expected voltage (Valid Battery Reading)/1
  Less than minimum threshold voltage (Battery level too low)/1 -> AND/2
  Greater than minimum expected voltage (Valid Battery Reading)/1 -> AND/1
  AND/1 -> Data Type Conversion/1
  Constant/1 -> Threshold/2
  Battery Low Time Threshold (s)/1 -> Threshold/3
  Data Type Conversion/1 -> Threshold/1
  Threshold/2 -> Terminator/1
  Threshold/1 -> Triggered Subsystem - Latching Flag/Trigger
  Triggered Subsystem - Latching Flag/1(Out1) -> Data Type Conversion1/1
  Data Type Conversion1/1 -> Low Battery/1

== system QD2_DroneStack_PID_AM32ESC_R2022b/QDrone 2 DAQ - OLD/Sensor Failure Monitoring ==
  note: Check if any of the IMU signal lines have "flatlined"
      | i.e., remain at exactly 0 value for 1 second or more
  IMU Data [12] : Inport
  Model Time : Inport  Port=2
  AND : Logic  IconShape=distinctive  AllPortsSameDT=off  OutDataTypeStr=boolean
  Compare : quarc_library/Logic Operations/Compare  operator=>=  output_data_type=boolean
      settings: SourceProductName=QUARC Targets
  Constant1 : Constant
  Constant2 : Constant  Value=0
  Demux : Demux  Outputs=12
  OR : Logic  Operator=OR  Inputs=12  AllPortsSameDT=off  OutDataTypeStr=boolean
  Terminator{,1..11} (12 alike) : Terminator
  Threshold{,1..11} (12 alike) : quarc_library/Discontinuities/Threshold  operator===  param_src=External input port  threshold=0  duration=1
      settings: SourceProductName=QUARC Targets
  Sensor Fault : Outport
  wires:
  Model Time/1 -> Compare/1
  Constant1/1 -> Threshold1/3, Threshold2/3, Threshold3/3, Threshold5/3, Threshold6/3, Threshold7/3, Threshold8/3, Threshold9/3, Threshold10/3, Threshold11/3, Threshold4/3, Threshold/3, Compare/2
  Demux/1 -> Threshold/1
  Demux/2 -> Threshold1/1
  Constant2/1 -> Threshold1/2, Threshold2/2, Threshold3/2, Threshold4/2, Threshold5/2, Threshold6/2, Threshold7/2, Threshold8/2, Threshold9/2, Threshold10/2, Threshold11/2, Threshold/2
  IMU Data [12]/1 -> Demux/1
  Demux/3 -> Threshold2/1
  Demux/4 -> Threshold3/1
  Demux/5 -> Threshold4/1
  Demux/6 -> Threshold5/1
  Demux/7 -> Threshold6/1
  Demux/8 -> Threshold7/1
  Demux/9 -> Threshold8/1
  Demux/10 -> Threshold9/1
  Demux/11 -> Threshold10/1
  Demux/12 -> Threshold11/1
  Threshold/1 -> OR/1
  Threshold1/1 -> OR/2
  Threshold2/1 -> OR/3
  Threshold3/1 -> OR/4
  Threshold4/1 -> OR/5
  Threshold5/1 -> OR/6
  Threshold6/1 -> OR/7
  Threshold7/1 -> OR/8
  Threshold8/1 -> OR/9
  Threshold9/1 -> OR/10
  Threshold10/1 -> OR/11
  Threshold11/1 -> OR/12
  Threshold/2 -> Terminator/1
  Threshold1/2 -> Terminator1/1
  Threshold2/2 -> Terminator2/1
  Threshold3/2 -> Terminator3/1
  Threshold4/2 -> Terminator4/1
  Threshold5/2 -> Terminator5/1
  Threshold6/2 -> Terminator6/1
  Threshold7/2 -> Terminator7/1
  Threshold8/2 -> Terminator8/1
  Threshold9/2 -> Terminator9/1
  Threshold10/2 -> Terminator10/1
  Threshold11/2 -> Terminator11/1
  Compare/1 -> AND/1
  OR/1 -> AND/2
  AND/1 -> Sensor Fault/1

== system QD2_DroneStack_PID_AM32ESC_R2022b/QDrone 2 DAQ - OLD/Timing Monitors ==
  note: Base Model Rate (1kHz)
  note: Optical Flow Rate (100 Hz)
  note: ToF Range Rate (25 Hz)
  Computation Time : quarc_library/Sources/Time/Computation Time  sample_time=qc_get_step_size  use_model=on  use_cpu_time=off
  Computation Time1 : quarc_library/Sources/Time/Computation Time  sample_time=0.01  use_model=on  use_cpu_time=off
  Computation Time2 : quarc_library/Sources/Time/Computation Time  sample_time=0.04  use_model=on  use_cpu_time=off
  Mux : Mux  Inputs=2
  Mux1 : Mux  Inputs=2
  Mux2 : Mux  Inputs=2
  Mux3 : Mux  Inputs=3
  Rate Transition{,1..3} (4 alike) : RateTransition
  Sample Time : quarc_library/Sources/Time/Sample Time  Priority=-99  sample_time=qc_get_step_size
  Sample Time1 : quarc_library/Sources/Time/Sample Time  Priority=-99  sample_time=0.01
  Sample Time2 : quarc_library/Sources/Time/Sample Time  Priority=-99  sample_time=0.04
  Timing Check : Scope  NumInputPorts=3
  Timings : Outport
  wires:
  Computation Time/1 -> Mux/1
  Sample Time/1 -> Mux/2
  Sample Time1/1 -> Rate Transition1/1
  Computation Time1/1 -> Rate Transition/1
  Computation Time2/1 -> Rate Transition2/1
  Sample Time2/1 -> Rate Transition3/1
  Mux1/1 -> Mux3/2, Timing Check/2
  Mux/1 -> Timing Check/1, Mux3/1
  Mux2/1 -> Timing Check/3, Mux3/3
  Mux3/1 -> Timings/1
  Rate Transition/1 -> Mux1/1
  Rate Transition1/1 -> Mux1/2
  Rate Transition2/1 -> Mux2/1
  Rate Transition3/1 -> Mux2/2

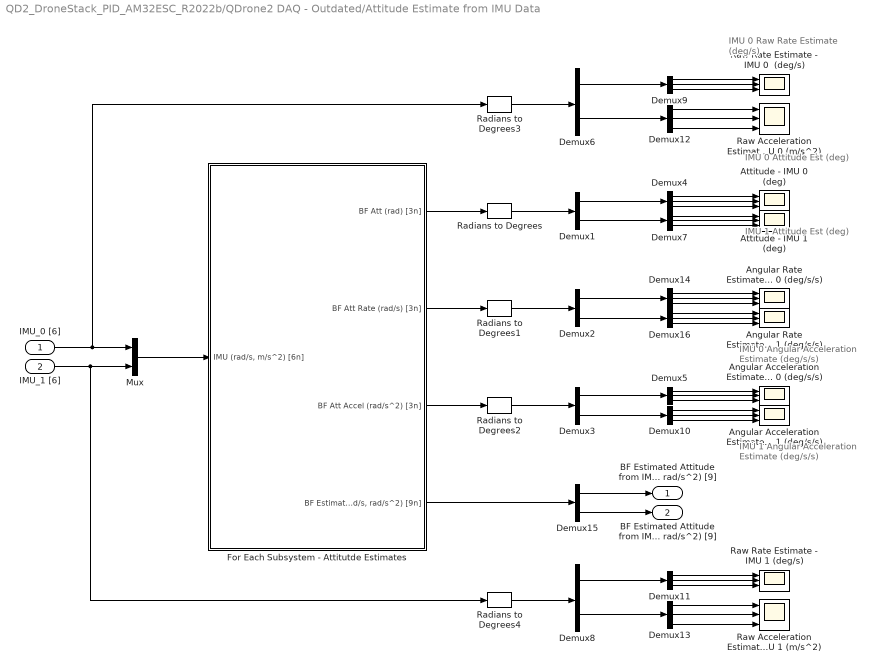
== system QD2_DroneStack_PID_AM32ESC_R2022b/QDrone2 DAQ - Outdated/Attitude Estimate from IMU Data ==
  note: IMU 0
      | Attitude Est (deg)
  note: IMU 1
      | Attitude Est (deg)
  note: IMU 0
      | Angular Acceleration
      | Estimate (deg/s/s)
  note: IMU 1
      | Angular Acceleration
      | Estimate (deg/s/s)
  note: IMU 0
      | Raw Rate Estimate (deg/s)
  IMU_0 [6] : Inport
  IMU_1 [6] : Inport  Port=2
  Angular Acceleration Estimate - IMU 0 (deg/s/s) : Scope  NumInputPorts=3
  Angular Acceleration Estimate IMU 1 (deg/s/s) : Scope  NumInputPorts=3
  Angular Rate Estimate - IMU 0 (deg/s/s) : Scope  NumInputPorts=3
  Angular Rate Estimate IMU 1 (deg/s/s) : Scope  NumInputPorts=3
  Attitude - IMU 0 (deg) : Scope  NumInputPorts=3
  Attitude - IMU 1 (deg) : Scope  NumInputPorts=3
  Demux{1..3,6,8} (5 alike) : Demux  Outputs=[3, 3]
  Demux{4..5,7,9..14,16} (10 alike) : Demux  Outputs=3
  Demux15 : Demux  Outputs=[9, 9]
  For Each Subsystem - Attitutde Estimates : Subsystem  TreatAsAtomicUnit=on
  Mux : Mux  Inputs=2
  Radians to Degrees{,1..4} (5 alike) : simulink_extras/Transformations/Radians to Degrees
  Raw Acceleration Estimate - IMU 0 (m/s^2) : Scope  NumInputPorts=3
  Raw Acceleration Estimate - IMU 1 (m/s^2) : Scope  NumInputPorts=3
  Raw Rate Estimate - IMU 0  (deg/s) : Scope  NumInputPorts=3
  Raw Rate Estimate - IMU 1 (deg/s) : Scope  NumInputPorts=3
  "BF Estimated Attitude from IMU 0 (rad, rad/s, rad/s^2) [9]" : Outport
  "BF Estimated Attitude from IMU 1 (rad, rad/s, rad/s^2) [9]" : Outport  Port=2
  wires:
  IMU_0 [6]/1 -> Radians to Degrees3/1, Mux/1
  IMU_1 [6]/1 -> Radians to Degrees4/1, Mux/2
  Mux/1 -> For Each Subsystem - Attitutde Estimates/1("IMU (rad/s, m/s^2) [6n]")
  For Each Subsystem - Attitutde Estimates/4("BF Estimated Att (rad, rad/s, rad/s^2) [9n] ") -> Demux15/1
  Demux15/1 -> "BF Estimated Attitude from IMU 0 (rad, rad/s, rad/s^2) [9]"/1
  Demux15/2 -> "BF Estimated Attitude from IMU 1 (rad, rad/s, rad/s^2) [9]"/1
  For Each Subsystem - Attitutde Estimates/1(BF Att (rad) [3n]) -> Radians to Degrees/1
  Radians to Degrees/1 -> Demux1/1
  For Each Subsystem - Attitutde Estimates/2(BF Att Rate (rad/s) [3n]) -> Radians to Degrees1/1
  For Each Subsystem - Attitutde Estimates/3(BF Att Accel (rad/s^2) [3n]) -> Radians to Degrees2/1
  Radians to Degrees1/1 -> Demux2/1
  Radians to Degrees2/1 -> Demux3/1
  Demux4/3 -> Attitude - IMU 0 (deg)/3
  Demux4/1 -> Attitude - IMU 0 (deg)/1
  Demux4/2 -> Attitude - IMU 0 (deg)/2
  Demux1/1 -> Demux4/1
  Demux7/2 -> Attitude - IMU 1 (deg)/2
  Demux7/1 -> Attitude - IMU 1 (deg)/1
  Demux7/3 -> Attitude - IMU 1 (deg)/3
  Demux1/2 -> Demux7/1
  Demux5/2 -> Angular Acceleration Estimate - IMU 0 (deg/s/s)/2
  Demux5/3 -> Angular Acceleration Estimate - IMU 0 (deg/s/s)/3
  Demux5/1 -> Angular Acceleration Estimate - IMU 0 (deg/s/s)/1
  Demux3/1 -> Demux5/1
  Demux10/1 -> Angular Acceleration Estimate IMU 1 (deg/s/s)/1
  Demux10/2 -> Angular Acceleration Estimate IMU 1 (deg/s/s)/2
  Demux10/3 -> Angular Acceleration Estimate IMU 1 (deg/s/s)/3
  Demux3/2 -> Demux10/1
  Demux12/2 -> Raw Acceleration Estimate - IMU 0 (m/s^2)/2
  Demux12/3 -> Raw Acceleration Estimate - IMU 0 (m/s^2)/3
  Demux12/1 -> Raw Acceleration Estimate - IMU 0 (m/s^2)/1
  Demux8/2 -> Demux13/1
  Demux13/2 -> Raw Acceleration Estimate - IMU 1 (m/s^2)/2
  Demux13/3 -> Raw Acceleration Estimate - IMU 1 (m/s^2)/3
  Demux13/1 -> Raw Acceleration Estimate - IMU 1 (m/s^2)/1
  Demux9/2 -> Raw Rate Estimate - IMU 0  (deg/s)/2
  Demux9/1 -> Raw Rate Estimate - IMU 0  (deg/s)/1
  Demux9/3 -> Raw Rate Estimate - IMU 0  (deg/s)/3
  Demux6/2 -> Demux12/1
  Demux6/1 -> Demux9/1
  Radians to Degrees3/1 -> Demux6/1
  Radians to Degrees4/1 -> Demux8/1
  Demux11/1 -> Raw Rate Estimate - IMU 1 (deg/s)/1
  Demux11/2 -> Raw Rate Estimate - IMU 1 (deg/s)/2
  Demux11/3 -> Raw Rate Estimate - IMU 1 (deg/s)/3
  Demux8/1 -> Demux11/1
  Demux2/2 -> Demux16/1
  Demux16/3 -> Angular Rate Estimate IMU 1 (deg/s/s)/3
  Demux16/1 -> Angular Rate Estimate IMU 1 (deg/s/s)/1
  Demux16/2 -> Angular Rate Estimate IMU 1 (deg/s/s)/2
  Demux2/1 -> Demux14/1
  Demux14/2 -> Angular Rate Estimate - IMU 0 (deg/s/s)/2
  Demux14/1 -> Angular Rate Estimate - IMU 0 (deg/s/s)/1
  Demux14/3 -> Angular Rate Estimate - IMU 0 (deg/s/s)/3

== system QD2_DroneStack_PID_AM32ESC_R2022b/QDrone2 DAQ - Outdated/Check Battery level ==
  Battery level : Inport
  Compare To Constant : simulink/Logic and Bit Operations/Compare To Constant  relop=<=  const=14  OutDataTypeStr=boolean
  Compare To Constant1 : simulink/Logic and Bit Operations/Compare To Constant  relop=>  const=0.5  OutDataTypeStr=boolean
  Data Type Conversion : DataTypeConversion  SaturateOnIntegerOverflow=off  RndMeth=Floor
  Data Type Conversion1 : DataTypeConversion  SaturateOnIntegerOverflow=off  RndMeth=Floor
  Logical Operator : Logic  AllPortsSameDT=off  OutDataTypeStr=boolean
  Terminator : Terminator
  Threshold : quarc_library/Discontinuities/Threshold  operator=>=  param_src=Specify via dialog  threshold=0.5  duration=0.3
      settings: SourceProductName=QUARC Targets
  Triggered Subsystem : Subsystem  TreatAsAtomicUnit=on
  Low Battery : Outport  VectorParamsAs1DForOutWhenUnconnected=off
  wires:
  Threshold/2 -> Terminator/1
  Battery level/1 -> Compare To Constant1/1, Compare To Constant/1
  Threshold/1 -> Logical Operator/2
  Logical Operator/1 -> Triggered Subsystem/Trigger
  Compare To Constant1/1 -> Logical Operator/1
  Compare To Constant/1 -> Data Type Conversion/1
  Data Type Conversion/1 -> Threshold/1
  Data Type Conversion1/1 -> Low Battery/1
  Triggered Subsystem/1(Out1) -> Data Type Conversion1/1

== system QD2_DroneStack_PID_AM32ESC_R2022b/QDrone2 DAQ - Outdated/Choose Motor Telemetry ==
  Bias1 : Bias  Bias=0:3  SaturateOnIntegerOverflow=off
  Constant : Constant  Value=[0 0 0 0; 0 0 0 1; 0 0 0 0; 0 0 1 0; 0 0 0 0; 0 1 0 0; 0 0 0 0; 1 0 0 0]
  Counter Free-Running : simulink/Sources/Counter Free-Running  NumBits=3  tsamp=-1
  Gain : Gain  Gain=.7
  Selector : Selector  NumberOfDimensions=2  IndexMode=Zero-based  InputPortWidth=3  IndexOptions=Index vector (port),Select all  Indices=[1 3],1  OutputSizes=1,1
  Telemetry : Scope
  Motor telemetry : Outport
  wires:
  Gain/1 -> Bias1/1
  Bias1/1 -> Telemetry/1
  Constant/1 -> Selector/1
  Counter Free-Running/1 -> Selector/2
  Selector/1 -> Motor telemetry/1, Gain/1

== system QD2_DroneStack_PID_AM32ESC_R2022b/QDrone2 DAQ - Outdated/Choose Motor Telemetry1 ==
  Channel : Inport
  Constant1 : Constant  Value=[1 0 0 0]
  Constant2 : Constant  Value=[0 1 0 0]
  Constant3 : Constant  Value=[0 0 1 0]
  Constant4 : Constant  Value=[0 0 0 1]
  Multiport Switch : MultiPortSwitch  DataPortOrder=Zero-based contiguous  Inputs=4  zeroidx=on  SaturateOnIntegerOverflow=off  InputSameDT=off
  Motor selection : Outport
  wires:
  Multiport Switch/1 -> Motor selection/1
  Constant4/1 -> Multiport Switch/5
  Constant3/1 -> Multiport Switch/4
  Constant1/1 -> Multiport Switch/2
  Constant2/1 -> Multiport Switch/3
  Channel/1 -> Multiport Switch/1

== system QD2_DroneStack_PID_AM32ESC_R2022b/QDrone2 DAQ - Outdated/Sensor Failure Monitoring - IMU0 ==
  note: Check for no data condition (flat-line zero) from any of the onboard sensors
  Sensor Data (rad/s,m/s^2)  [6] : Inport
  Data Type Conversion1 : DataTypeConversion  SaturateOnIntegerOverflow=off  RndMeth=Floor
  Data Type Conversion2 : DataTypeConversion  SaturateOnIntegerOverflow=off  RndMeth=Floor
  Data Type Conversion4 : DataTypeConversion  SaturateOnIntegerOverflow=off  RndMeth=Floor
  Demux : Demux  Outputs=[3 3]
  Logical Operator : Logic  Operator=OR  Inputs=1  AllPortsSameDT=off  OutDataTypeStr=boolean
  Mux : Mux  Inputs=2
  Sensor Failure (Accelerometer) : Subsystem
  Sensor Failure (Gyroscope) : Subsystem
  IMU Failure : Outport  VectorParamsAs1DForOutWhenUnconnected=off
  wires:
  Data Type Conversion4/1 -> IMU Failure/1
  Logical Operator/1 -> Data Type Conversion4/1
  Demux/1 -> Sensor Failure (Gyroscope)/1(Sensor Input)
  Data Type Conversion1/1 -> Mux/2
  Data Type Conversion2/1 -> Mux/1
  Mux/1 -> Logical Operator/1
  Sensor Failure (Accelerometer)/1(Sensor Fault) -> Data Type Conversion1/1
  Sensor Failure (Gyroscope)/1(Sensor Fault) -> Data Type Conversion2/1
  Demux/2 -> Sensor Failure (Accelerometer)/1(Sensor Input)
  Sensor Data (rad/s,m/s^2)  [6]/1 -> Demux/1

== system QD2_DroneStack_PID_AM32ESC_R2022b/QDrone2 DAQ - Outdated/Sensor Failure Monitoring - IMU1 ==
  note: Check for no data condition (flat-line zero) from any of the onboard sensors
  Sensor Data (rad/s,m/s^2)  [6] : Inport
  Data Type Conversion1 : DataTypeConversion  SaturateOnIntegerOverflow=off  RndMeth=Floor
  Data Type Conversion2 : DataTypeConversion  SaturateOnIntegerOverflow=off  RndMeth=Floor
  Data Type Conversion4 : DataTypeConversion  SaturateOnIntegerOverflow=off  RndMeth=Floor
  Demux : Demux  Outputs=[3 3]
  Logical Operator : Logic  Operator=OR  Inputs=1  AllPortsSameDT=off  OutDataTypeStr=boolean
  Mux : Mux  Inputs=2
  Sensor Failure (Accelerometer) : Subsystem
  Sensor Failure (Gyroscope) : Subsystem
  IMU Failure : Outport  VectorParamsAs1DForOutWhenUnconnected=off
  wires:
  Sensor Data (rad/s,m/s^2)  [6]/1 -> Demux/1
  Demux/2 -> Sensor Failure (Accelerometer)/1(Sensor Input)
  Sensor Failure (Gyroscope)/1(Sensor Fault) -> Data Type Conversion2/1
  Sensor Failure (Accelerometer)/1(Sensor Fault) -> Data Type Conversion1/1
  Mux/1 -> Logical Operator/1
  Data Type Conversion2/1 -> Mux/1
  Data Type Conversion1/1 -> Mux/2
  Demux/1 -> Sensor Failure (Gyroscope)/1(Sensor Input)
  Logical Operator/1 -> Data Type Conversion4/1
  Data Type Conversion4/1 -> IMU Failure/1

== system QD2_DroneStack_PID_AM32ESC_R2022b/QDrone2 DAQ - Outdated/Subsystem ==
  note: PCB LED 2
  note: PCB LED 1
  E_Stop (0,1) : Inport
  "Arm(0,1) " : Inport  Port=2
  Battery_State (bool) : Inport  Port=3
  Blue : Constant  Value=[0 0 1]
  Green : Constant  Value=[0 1 0]
  MATLAB Function LED Color Assignment : MATLAB Function  TreatAsAtomicUnit=on
  Multiport Switch : MultiPortSwitch  SaturateOnIntegerOverflow=off  InputSameDT=off
  Mux : Mux  Inputs=2
  Red : Constant  Value=[1 0 0]
  LEDs(%) [6] : Outport
  wires:
  Mux/1 -> LEDs(%) [6]/1
  Multiport Switch/1 -> Mux/1, Mux/2
  Blue/1 -> Multiport Switch/4
  Green/1 -> Multiport Switch/3
  Red/1 -> Multiport Switch/2
  Battery_State (bool)/1 -> MATLAB Function LED Color Assignment/3(low_battery)
  E_Stop (0,1)/1 -> MATLAB Function LED Color Assignment/1(E_Stop)
  "Arm(0,1) "/1 -> MATLAB Function LED Color Assignment/2(Arm)
  MATLAB Function LED Color Assignment/1(value) -> Multiport Switch/1

== system QD2_DroneStack_PID_AM32ESC_R2022b/QDrone2 DAQ - Outdated/Subsystem1 ==
  ESC % : Inport
  Motor command : Inport  Port=2
  Demux1 : Demux
  Demux3 : Demux
  Maintain previous value4 : Subsystem
  Mux{,1..3} (4 alike) : Mux  Inputs=2
  Selector : Selector  InputPortWidth=4  IndexOptions=Index vector (dialog)  Indices=[4 3 2 1]  OutputSizes=1
  Selector1 : Selector  InputPortWidth=4  IndexOptions=Index vector (dialog)  Indices=[4 3 2 1]  OutputSizes=1
  Out1 : Outport
  Out2 : Outport  Port=2
  Out3 : Outport  Port=3
  Out4 : Outport  Port=4
  wires:
  Motor command/1 -> Selector/1
  Demux1/2 -> Mux1/1
  Selector/1 -> Demux1/1
  Demux1/1 -> Mux/1
  Demux1/4 -> Mux3/1
  Demux1/3 -> Mux2/1
  Mux3/1 -> Out4/1
  Mux2/1 -> Out3/1
  Mux/1 -> Out1/1
  Mux1/1 -> Out2/1
  ESC %/1 -> Selector1/1
  Demux3/1 -> Mux/2
  Demux3/2 -> Mux1/2
  Demux3/3 -> Mux2/2
  Demux3/4 -> Mux3/2
  Selector1/1 -> Maintain previous value4/1(Value in)
  Maintain previous value4/1(Non 0 values) -> Demux3/1
